simulink model "TECSHarness"  (R2023a)
settings: Solver=ode4  StartTime=0.0  StopTime=t(end)  FixedStep=dt  RelTol=1e-3
undefined symbols (not defined in the file): dt, Pitch, TECS, TO
libraries: Actuators x1, PitchController x1, TECSController x1, Telemaster_Lib x1
settings Model: Creator=igmso  LastModifiedBy=igmso
settings DataIOCC: ExternalInput=[t,u]  InitialState=getstatestruct(SteadyState(idx).op)  SaveFormat=StructureWithTime

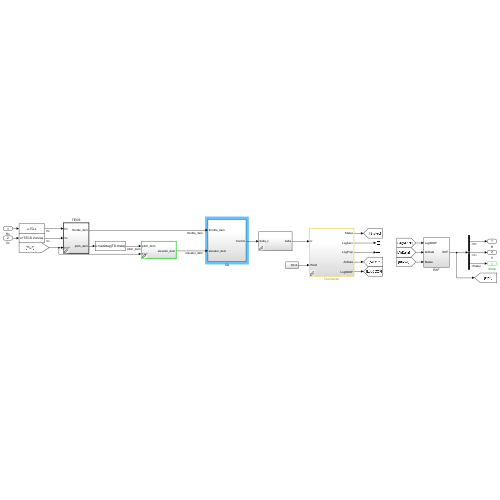
[thumbnail: Simulink's stored preview of the top-level diagram]
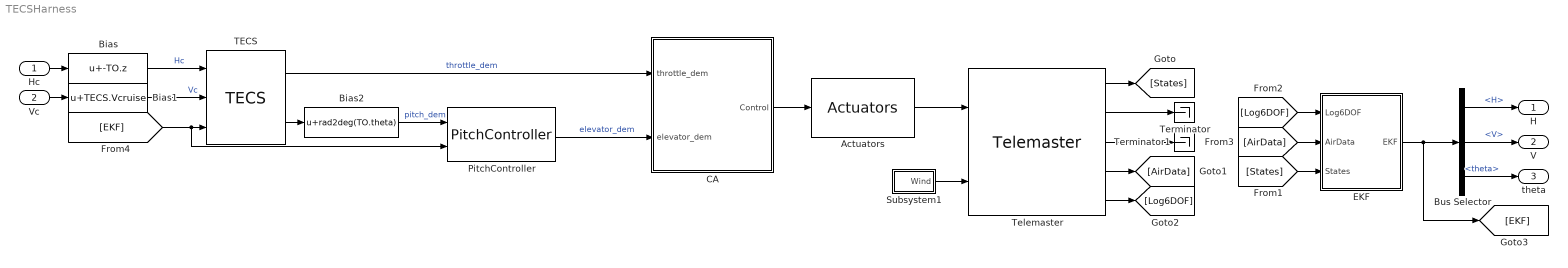
== system TECSHarness ==
  Hc : Inport  SampleTime=1/TECS.ControlRate
  Vc : Inport  Port=2  SampleTime=1/TECS.ControlRate
  Actuators : Actuators/Actuators  SystemSampleTime=-1  VariantActivationTime=update diagram  Latency=0  AutoFrameSizeCalculation=off
  Bias : Bias  Bias=-TO.z  SaturateOnIntegerOverflow=off
  Bias1 : Bias  Bias=TECS.Vcruise  SaturateOnIntegerOverflow=off
  Bias2 : Bias  Bias=rad2deg(TO.theta)  SaturateOnIntegerOverflow=off
  Bus Selector : BusSelector  OutputSignals=H,V,States.theta
  CA : Subsystem
  EKF : Subsystem
  PitchController : PitchController/PitchController  SystemSampleTime=1/Pitch.ControlRate  VariantActivationTime=update diagram  Latency=0  AutoFrameSizeCalculation=off
  Subsystem1 : Subsystem
  TECS : TECSController/TECS  SystemSampleTime=-1  VariantActivationTime=update diagram  Latency=0  AutoFrameSizeCalculation=off
  Telemaster : Telemaster_Lib/Telemaster  SystemSampleTime=-1  VariantActivationTime=update diagram  Latency=0  AutoFrameSizeCalculation=off
  Terminator : Terminator
  Terminator1 : Terminator
  H : Outport
  V : Outport  Port=2
  theta : Outport  Port=3
  wires:
  Telemaster/1 -> [States]
  Telemaster/4 -> [AirData]
  Telemaster/2 -> Terminator/1
  Telemaster/3 -> Terminator1/1
  Subsystem1/1(Wind) -> Telemaster/2
  [Log6DOF] -> EKF/1(Log6DOF)
  [AirData] -> EKF/2(AirData)
  EKF/1(EKF) -> Bus Selector/1, [EKF]
  [States] -> EKF/3(States)
  Telemaster/5 -> [Log6DOF]
  TECS/2 -> Bias2/1
  [EKF] -> PitchController/2, TECS/3
  Bias/1 -> TECS/1  "Hc"
  Bias1/1 -> TECS/2  "Vc"
  Bus Selector/1 -> H/1  "<H>"
  Bus Selector/2 -> V/1  "<V>"
  Bus Selector/3 -> theta/1  "<theta>"
  Vc/1 -> Bias1/1
  Bias2/1 -> PitchController/1  "pitch_dem"
  Hc/1 -> Bias/1
  TECS/1 -> CA/1(throttle_dem)  "throttle_dem"
  PitchController/1 -> CA/2(elevator_dem)  "elevator_dem"
  CA/1(Control) -> Actuators/1
  Actuators/1 -> Telemaster/1

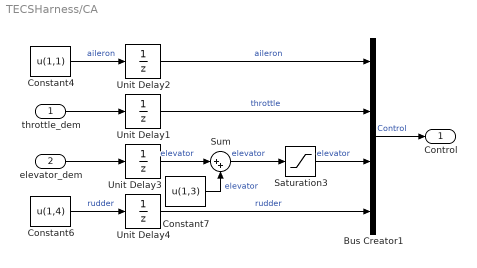
== system TECSHarness/CA ==
  throttle_dem : Inport
  elevator_dem : Inport  Port=2
  Bus Creator1 : BusCreator  Inputs=4
  Constant4 : Constant  Value=u(1,1)  SampleTime=1/400
  Constant6 : Constant  Value=u(1,4)  SampleTime=1/400
  Constant7 : Constant  Value=u(1,3)  SampleTime=1/400
  Saturation3 : Saturate  UpperLimit=20  LowerLimit=-20
  Sum : Sum  Inputs=|++
  Unit Delay1 : UnitDelay  InitialCondition=u(1,2)  SampleTime=1/400  StateName=elevator_CA  HasFrameUpgradeWarning=on
  Unit Delay2 : UnitDelay  InitialCondition=u(1,2)  SampleTime=1/400  StateName=elevator_CA  HasFrameUpgradeWarning=on
  Unit Delay3 : UnitDelay  SampleTime=1/400  StateName=elevator_CA  HasFrameUpgradeWarning=on
  Unit Delay4 : UnitDelay  InitialCondition=u(1,2)  SampleTime=1/400  StateName=elevator_CA  HasFrameUpgradeWarning=on
  Control : Outport
  wires:
  Sum/1 -> Saturation3/1  "elevator"
  Unit Delay4/1 -> Bus Creator1/4  "rudder"
  Constant4/1 -> Unit Delay2/1  "aileron"
  Saturation3/1 -> Bus Creator1/3  "elevator"
  Constant6/1 -> Unit Delay4/1  "rudder"
  Unit Delay3/1 -> Sum/1  "elevator"
  Constant7/1 -> Sum/2  "elevator"
  elevator_dem/1 -> Unit Delay3/1
  Unit Delay1/1 -> Bus Creator1/2  "throttle"
  Unit Delay2/1 -> Bus Creator1/1  "aileron"
  throttle_dem/1 -> Unit Delay1/1
  Bus Creator1/1 -> Control/1  "Control"

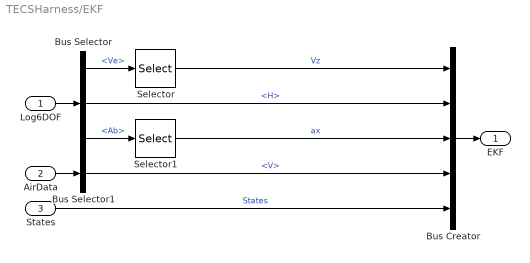
== system TECSHarness/EKF ==
  Log6DOF : Inport  SampleTime=1/400
  AirData : Inport  Port=2  SampleTime=1/400
  States : Inport  Port=3  SampleTime=1/400
  Bus Selector : BusSelector  OutputSignals=Ve,H,Ab
  Bus Selector1 : BusSelector  OutputSignals=V
  Bus Creator : BusCreator  Inputs=5
  Selector : Selector  InputPortWidth=3  IndexOptions=Index vector (dialog)  Indices=3  OutputSizes=1
  Selector1 : Selector  InputPortWidth=3  IndexOptions=Index vector (dialog)  Indices=1  OutputSizes=1
  EKF : Outport  SampleTime=1/400
  wires:
  Bus Selector/1 -> Selector/1  "<Ve>"
  Selector1/1 -> Bus Creator/3  "ax"
  Bus Selector/3 -> Selector1/1  "<Ab>"
  Log6DOF/1 -> Bus Selector/1
  Bus Selector1/1 -> Bus Creator/4  "<V>"
  Bus Selector/2 -> Bus Creator/2  "<H>"
  AirData/1 -> Bus Selector1/1
  Bus Creator/1 -> EKF/1
  Selector/1 -> Bus Creator/1  "Vz"
  States/1 -> Bus Creator/5  "States"

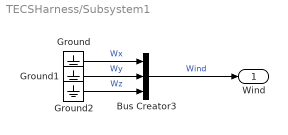
== system TECSHarness/Subsystem1 ==
  Bus Creator3 : BusCreator  Inputs=3
  Ground : Ground
  Ground1 : Ground
  Ground2 : Ground
  Wind : Outport  SampleTime=dt
  wires:
  Ground1/1 -> Bus Creator3/2  "Wy"
  Ground2/1 -> Bus Creator3/3  "Wz"
  Bus Creator3/1 -> Wind/1  "Wind"
  Ground/1 -> Bus Creator3/1  "Wx"
